simulink model "ControllerModeSelector"  (R2024a)
settings: configuration reference "csMultiInstance" (kept outside this file)
undefined symbols (not defined in the file or in its folder): BrStatus, Default_decel, FB_decel, max_ac, max_dc, min_ac, Ts
Description:
  | Model to output acceleration based on information from the MPC and Watchdog controller. This is considered as a SW unit.
settings Model: DataDictionary=DD_ControllerModeSelector.sldd  EnableAccessToBaseWorkspace=off  Creator=The MathWorks, Inc.  LastModifiedBy=The MathWorks, Inc.
settings ConfigSetRef: SourceName=csMultiInstance

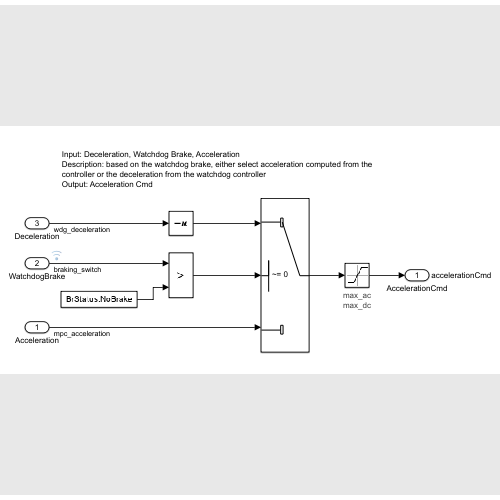
[thumbnail: Simulink's stored preview of the top-level diagram]
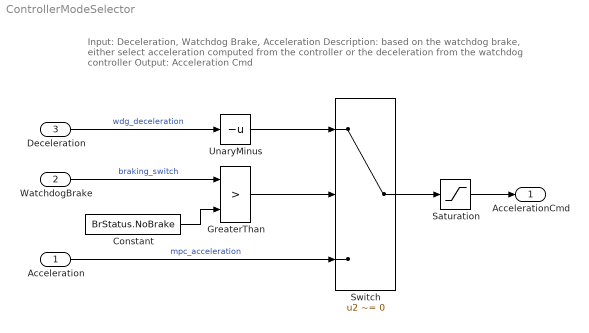
== system ControllerModeSelector ==
  note: Input: Deceleration, Watchdog Brake, Acceleration
      | Description: based on the watchdog brake, either select acceleration computed from the controller or the deceleration from the watchdog controller
      | Output: Acceleration Cmd
  Acceleration : Inport  OutMin=min_ac-1  OutMax=max_ac  OutDataTypeStr=Acceleration_DType  Unit=m/s^2  PortDimensions=Acceleration_Dimensions  SampleTime=Ts
  WatchdogBrake : Inport  Port=2  OutDataTypeStr=Enum: BrStatus  PortDimensions=BrStatus_Dimensions  SampleTime=Ts
  Deceleration : Inport  Port=3  OutMin=Default_decel  OutMax=FB_decel  OutDataTypeStr=Acceleration_DType  Unit=m/s^2  PortDimensions=Acceleration_Dimensions  SampleTime=Ts
  Constant : Constant  Value=BrStatus.NoBrake  OutDataTypeStr=Enum: BrStatus
  GreaterThan : RelationalOperator  Operator=>  RndMeth=Simplest  InputSameDT=off
  Saturation : Saturate  UpperLimit=max_ac  LowerLimit=max_dc
      settings: AttributesFormatString=|
      | %<UpperLimit>
      | %<LowerLimit>
  Switch : Switch  Criteria=u2 ~= 0  SaturateOnIntegerOverflow=off  InputSameDT=off
  UnaryMinus : UnaryMinus  SaturateOnIntegerOverflow=on
  AccelerationCmd : Outport  SignalName=accelerationCmd  OutMin=max_dc  OutMax=max_ac  OutDataTypeStr=Acceleration_DType  Unit=m/s^2  PortDimensions=Acceleration_Dimensions  SampleTime=Ts  VectorParamsAs1DForOutWhenUnconnected=off
  wires:
  Switch/1 -> Saturation/1
  Saturation/1 -> AccelerationCmd/1
  Deceleration/1 -> UnaryMinus/1  "wdg_deceleration"
  UnaryMinus/1 -> Switch/1
  Acceleration/1 -> Switch/3  "mpc_acceleration"
  WatchdogBrake/1 -> GreaterThan/1  "braking_switch"
  GreaterThan/1 -> Switch/2
  Constant/1 -> GreaterThan/2
